simulink model "diaforiko_epitaxinsh_PID_test_v4"  (R2024b)
settings: Solver=FixedStepDiscrete  StartTime=0.0  StopTime=10.0  FixedStep=0.02  RelTol=1e-3  EnableMultiTasking=on
libraries: frdmtfcshieldlib x6, Autonomous_Vehicle_Competition x1
settings Model: ExtModeTrigDuration=5  Creator=akrdi  LastModifiedBy=kapki
settings SolverCC: AutoInsertRateTranBlk=on
settings OptimizationCC: EnhancedBackFolding=on  PassReuseOutputArgsThreshold=0  MaxStackSize=64  OptimizeBlockOrder=speed  DifferentSizesBufferReuse=on  OptimizationCustomize=off
settings DebuggingCC: ParameterTunabilityLossMsg=error
settings HardwareCC: ProdBitPerPointer=32  ProdBitPerSizeT=32  ProdBitPerPtrDiffT=32  ProdLargestAtomicInteger=Long  ProdLargestAtomicFloat=Double  ProdWordSize=32  ProdHWDeviceType=ARM Compatible->ARM Cortex  UseEmbeddedCoderFeatures=off
settings SFSimCC: MATLABDynamicMemAlloc=off
settings RTWCC: Description=Embedded Coder  SystemTargetFile=ert.tlc  HardwareBoard=NXP FRDM-KL25Z  TemplateMakefile=ert_default_tmf  Toolchain=GNU Tools for ARM Embedded Processors  GPUComputeCapability=3.5
settings CodeAppCC: ForceParamTrailComments=on  OperatorAnnotations=on
settings ERTTargetCC: ERTCustomFileBanners=off  SupportContinuousTime=on  SupportNonInlinedSFcns=on  RemoveResetFunc=off  ModelStepFunctionPrototypeControlCompliant=off  ExtModeTransport=1  ExtModeMexFile=ext_serial_win32_comm  InlinedParameterPlacement=Hierarchical  DynamicArrayContainerType=coder::array

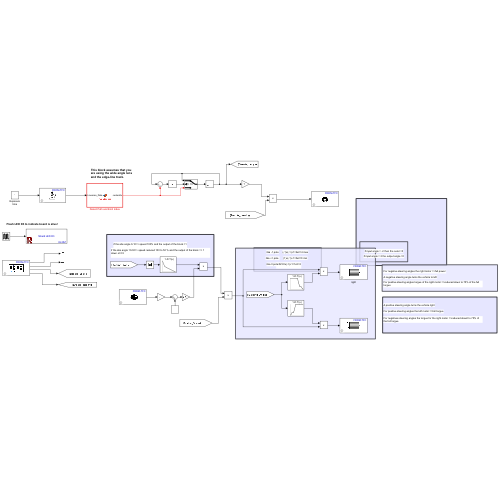
[thumbnail: Simulink's stored preview of the top-level diagram]
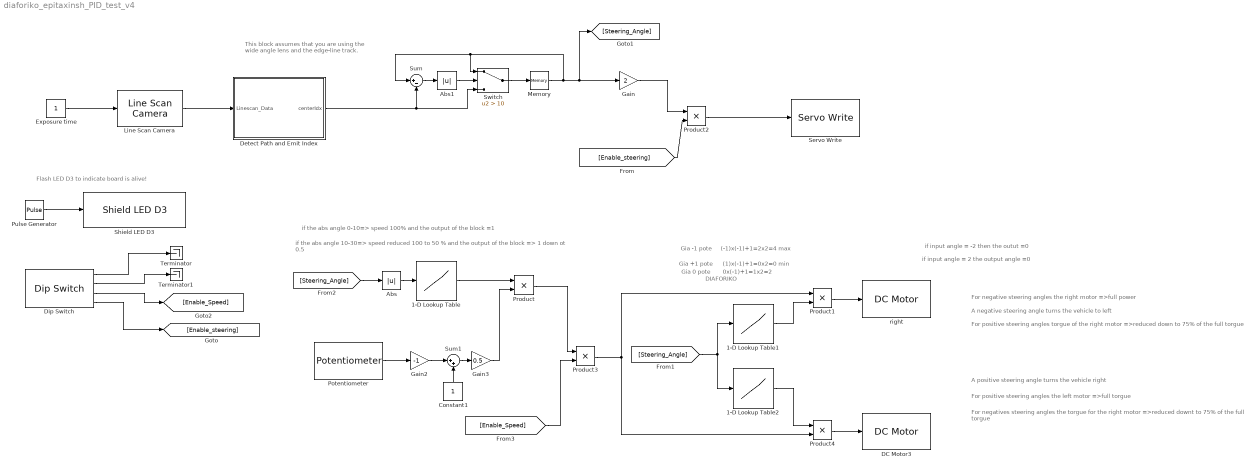
== system diaforiko_epitaxinsh_PID_test_v4 ==
  note: if the abs angle 0-10=> speed 100% and the output of the block =1
  note: Flash LED D3 to indicate board is alive!
  note: A positive steering angle turns the vehicle right
  note: For negatives steering angles the torgue for the right motor =>reduced downt to 75% of the full torgue
  note: This block assumes that you are using the wide angle lens
      | and the edge-line track.
  note: For positive steering angles the left motor =>full torgue
  note: if the abs angle 10-30=> speed reduced 100 to 50 % and the output of the block => 1 down ot 0.5
  note: For positive steering angles torgue of the right motor =>reduced down to 75% of the full torgue
  note: A negative steering angle turns the vehicle to left
  note: DIAFORIKO
  note: For negative steering angles the right motor =>full power
  note: 0x(-1)+1=1x2=2
  note: Gia +1 pote
  note: (1)x(-1)+1=0x2=0 min
  note: Gia -1 pote
  note: Gia 0 pote
  note: if input angle = 2 the output angle =0
  note: if input angle = -2 then the outut =0
  note: (-1)x(-1)+1=2x2=4 max
  1-D Lookup Table : Lookup_n-D  NumberOfTableDimensions=1  BreakpointsForDimension1=[0 10 20 60]  Table=[1.8 1 0.8 0.2]  ExtrapMethod=Clip  UseLastTableValue=on  InternalRulePriority=Speed  RndMeth=Simplest
  1-D Lookup Table1 : Lookup_n-D  NumberOfTableDimensions=1  BreakpointsForDimension1=[ -70 0 10 20 30 35 40 50 60 70]  Table="[1 1  1 0.77 0.65 0.58 0.57 0.57 0.50 0.45 ]"  ExtrapMethod=Clip  UseLastTableValue=on  InternalRulePriority=Speed  RndMeth=Simplest
  1-D Lookup Table2 : Lookup_n-D  NumberOfTableDimensions=1  BreakpointsForDimension1=[ -70 -60 -50 -40 -35 -30 -20 -10 0 10 20 30 35 40 50 60 70]  Table=[0.45 0.5 0.57 0.57 0.58 0.65 0.77 1 1 1 1 1 1 1 1 1 1]  ExtrapMethod=Clip  UseLastTableValue=on  InternalRulePriority=Speed  RndMeth=Simplest
  Abs : Abs  SaturateOnIntegerOverflow=off
  Abs1 : Abs  SaturateOnIntegerOverflow=off
  Constant1 : Constant
  DC Motor3 : frdmtfcshieldlib/DC Motor  WhichMotor=B
  Detect Path and Emit Index : MATLAB Function  TreatAsAtomicUnit=on
  Dip Switch : frdmtfcshieldlib/Dip Switch  SampleTime=-1
  Exposure time : Constant
  Gain : Gain  Gain=2
  Gain2 : Gain  Gain=-1
  Gain3 : Gain  Gain=0.5
  Line Scan Camera : frdmtfcshieldlib/Line Scan Camera  CameraHeader=0  SampleTime=.02
  Memory : Memory  InitialCondition=64
  Potentiometer : frdmtfcshieldlib/Potentiometer  WhichPot=B  SampleTime=-1
  Product{,1..4} (5 alike) : Product
  Pulse Generator : DiscretePulseGenerator  PulseType=Time based  Period=10  PulseWidth=5
  Servo Write : frdmtfcshieldlib/Servo Write  WhichServo=0  minAngle=-30  maxAngle=30
  Shield LED D3 : Autonomous_Vehicle_Competition/Shield LED D3
      settings: SourceProductName=Autonomous Vehicle Competition
  Sum : Sum  Inputs=|+-
  Sum1 : Sum  Inputs=|++
  Switch : Switch  Criteria=u2 > Threshold  Threshold=10  SaturateOnIntegerOverflow=off  InputSameDT=off
  Terminator : Terminator
  Terminator1 : Terminator
  right : frdmtfcshieldlib/DC Motor  WhichMotor=A
  wires:
  [Enable_Speed] -> Product3/2
  Product4/1 -> DC Motor3/1
  Potentiometer/1 -> Gain2/1
  Product2/1 -> Servo Write/1
  [Steering_Angle] -> Abs/1
  Exposure time/1 -> Line Scan Camera/1
  1-D Lookup Table2/1 -> Product4/1
  Product/1 -> Product3/1
  Sum1/1 -> Gain3/1
  Product1/1 -> right/1
  [Steering_Angle] -> 1-D Lookup Table2/1, 1-D Lookup Table1/1
  Line Scan Camera/1 -> Detect Path and Emit Index/1(Linescan_Data)
  Product3/1 -> Product1/1, Product4/2
  Gain3/1 -> Product/2
  Dip Switch/1 -> Terminator/1
  Abs/1 -> 1-D Lookup Table/1
  [Enable_steering] -> Product2/2
  Constant1/1 -> Sum1/2
  Dip Switch/2 -> Terminator1/1
  Pulse Generator/1 -> Shield LED D3/1
  1-D Lookup Table/1 -> Product/1
  Dip Switch/3 -> [Enable_Speed]
  Gain2/1 -> Sum1/1
  1-D Lookup Table1/1 -> Product1/2
  Dip Switch/4 -> [Enable_steering]
  Gain/1 -> Product2/1
  Detect Path and Emit Index/1(centerIdx) -> Switch/3, Sum/2
  Sum/1 -> Abs1/1
  Abs1/1 -> Switch/2
  Switch/1 -> Memory/1
  Memory/1 -> [Steering_Angle], Gain/1, Switch/1, Sum/1

== matlab function diaforiko_epitaxinsh_PID_test_v4/Detect Path and Emit Index ==
  data: centerIdx output single; Linescan_Data input
function centerIdx = CenterIdx(Linescan_Data)
% function centerIdx = CenterIdx(Linescan_Data)
% This function finds the current position of the track's
% center. 

%%---------------------------------------------------------------------------------------------
% The lines below are also inside  file "Full_High_School_Model_0_View_Camera.m"
% This m-file will display the camera data and also the edges and center of
% the track using the same algorithm the vehicle uses. If you modify the
% lines below, you must also modify the same lines in file
% "Full_High_School_Model_0_View_Camera.m".
% 

First_Edge=single(1);
Second_Edge=single(128);

% Calculate the threshold as 75% of the mean value of the bright section of
% the track.
Threshold=0.75*mean(Linescan_Data(40:80));

%Find the First Edge
for i=64:-1:2
    if Linescan_Data(i)<Threshold
        First_Edge=single(i);
        break;
    end
end

% Find the Second Edge
for i=64:1:127
    if Linescan_Data(i)<Threshold
        Second_Edge=single(i);
        break;
    end
end

% If the edge indices are valid, then calculate the 
% center as the average of the two edge indices.
if First_Edge>1 && Second_Edge<128
    centerIdx=(Second_Edge+First_Edge)/2;
else
    centerIdx=single(255);
end

%Paste changes to the lines above in inside  file "Full_High_School_Model_0_View_Camera.m"
%----------------------------------------------------------------------------------------------------------


%%end  minimum finding algorithm

end
